simulink model "multirateFilters"  (R2017b)
settings: Solver=FixedStepDiscrete  StartTime=0.0  StopTime=0.02  RelTol=1e-3
undefined symbols (not defined in the file): designMultirateFIR
libraries: dspsrcs4 x4, dsparch4 x2, dspmlti4 x2, dspfdesign x1, dspsigops x1
settings Model: Creator=Lucas  LastModifiedBy=Lucas
settings SolverCC: AutoInsertRateTranBlk=on
settings DataIOCC: LimitDataPoints=on  SaveOutput=off  SignalLogging=off  SaveTime=off
settings OptimizationCC: LifeSpan=inf  SimCompilerOptimization=on
settings DebuggingCC: AlgebraicLoopMsg=error  SingleTaskRateTransMsg=error  AllowSymbolicDim=off  SFUnexpectedBacktrackingDiag=warning  SFNoUnconditionalDefaultTransitionDiag=warning  SFExecutionAtInitializationDiag=none
settings CodeAppCC: StateflowObjectComments=on
settings GRTTargetCC: TargetLangStandard=C89/C90 (ANSI)  GeneratePreprocessorConditionals=Disable all
settings ConfigComp: CovMetricSettings=dw  CovHtmlReporting=on  CovSaveCumulativeToWorkspaceVar=on  CovSaveSingleToWorkspaceVar=on  CovExternalEMLEnable=off  CovSFcnEnable=off

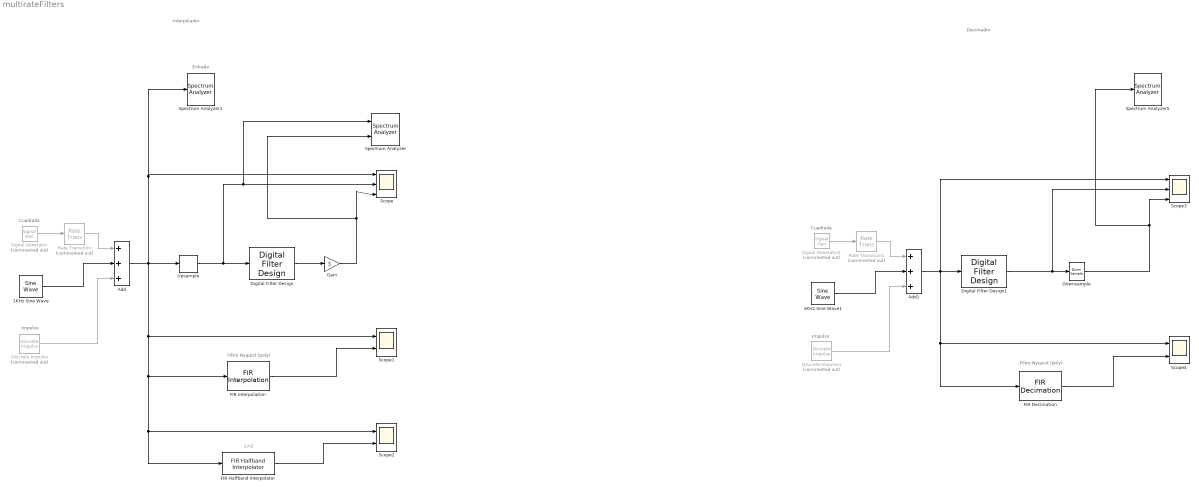
== system multirateFilters ==
  note: Interpolador
  note: Filtro Nyquist (poly)
  note: Entrada
  note: Cuadrada
  note: Filtro Nyquist (poly)
  note: Cuadrada
  note: Decimador
  note: Impulso
  note: Impulso
  note: L=2
  1KHz Sine Wave : dspsrcs4/Sine Wave  Amplitude=1  Frequency=1000  Phase=0  SampleMode=Discrete  OutComplex=Real  CompMethod=Trigonometric fcn  TableSize=Speed  SampleTime=1/10000  SamplesPerFrame=256  ResetState=Restart at time zero  OutputFrames=off  dataType=double  wordLen=16  udDataType=sfix(16)  fracBitsMode=Best precision  numFracBits=15  OutDataTypeStr=double  LastOutDataTypeStr=double
  1KHz Sine Wave1 : dspsrcs4/Sine Wave  Amplitude=1  Frequency=1000  Phase=0  SampleMode=Discrete  OutComplex=Real  CompMethod=Trigonometric fcn  TableSize=Speed  SampleTime=1/10000  SamplesPerFrame=300  ResetState=Restart at time zero  OutputFrames=off  dataType=double  wordLen=16  udDataType=sfix(16)  fracBitsMode=Best precision  numFracBits=15  OutDataTypeStr=double  LastOutDataTypeStr=double
  Add : Sum  Inputs=+++
  Add1 : Sum  Inputs=+++
  Digital Filter Design : dsparch4/Digital Filter Design  mwdsp_browser_bugfix_var=off
  Digital Filter Design1 : dsparch4/Digital Filter Design  mwdsp_browser_bugfix_var=off
  Discrete Impulse : dspsrcs4/Discrete  Impulse  Commented=on  Delay=0  SampleTime=1/10000  FrameSample=256  OutputFrames=off  dataType=double  isSigned=on  wordLen=16  udDataType=sfix(16)  fracBitsMode=Best precision  numFracBits=15  OutDataTypeStr=double  LastOutDataTypeStr=double
  Discrete Impulse1 : dspsrcs4/Discrete  Impulse  Commented=on  Delay=0  SampleTime=1/10000  FrameSample=300  OutputFrames=off  dataType=double  isSigned=on  wordLen=16  udDataType=sfix(16)  fracBitsMode=Best precision  numFracBits=15  OutDataTypeStr=double  LastOutDataTypeStr=double
  Downsample : DownSample  N=3
  FIR Decimation : dspmlti4/FIR Decimation  FilterSource=Auto  h=designMultirateFIR(1,2)  D=3  filtStruct=Direct form  FilterObject=FDECIM  InputProcessing=Columns as channels (frame based)  framing=Enforce single-rate processing  inputOffset=0  outputBufInitCond=0  roundingMode=Floor  overflowMode=off  firstCoeffDataTypeStr=Inherit: Same word length as input  firstCoeffMin=[]  firstCoeffMax=[]  firstCoeffLastDataTypeStr=Inherit: Same word length as input  outputDataTypeStr=Inherit: Same as accumulator  outputMin=[]  outputMax=[]  outputLastDataTypeStr=Inherit: Same as accumulator
  FIR Interpolation : dspmlti4/FIR Interpolation  FilterSource=Auto  h=designMultirateFIR(3,1)  L=3  FilterObject=FINTERP  InputProcessing=Columns as channels (frame based)  framing=Enforce single-rate processing  outputBufInitCond=0  roundingMode=Floor  overflowMode=off  firstCoeffDataTypeStr=Inherit: Same word length as input  firstCoeffMin=[]  firstCoeffMax=[]  firstCoeffLastDataTypeStr=Inherit: Same word length as input  outputDataTypeStr=Inherit: Same as accumulator  outputMin=[]  outputMax=[]  outputLastDataTypeStr=Inherit: Same as accumulator
      settings: SourceProductName=DSP System Toolbox
  FIR Halfband Interpolator : dspfdesign/FIR Halfband Interpolator  Specification=Transition width and stopband attenuation  FilterOrder=52  TransitionWidth=5000  StopbandAttenuation=80  FilterBankInputPort=off  InheritSampleRate=off  SampleRate=10000  SimulateUsing=Code generation  roundingMode=Floor  coeffsDataTypeStr=fixdt(1,16)
      settings: SourceProductName=DSP System Toolbox  SourceProductBaseCode=DS
  Gain : Gain  Gain=3
  Rate Transition : RateTransition  Commented=on
  Rate Transition1 : RateTransition  Commented=on
  Scope : Scope  NumInputPorts=3
  Scope1 : Scope  NumInputPorts=2
  Scope2 : Scope  NumInputPorts=2
  Scope3 : Scope  NumInputPorts=3
  Scope4 : Scope  NumInputPorts=2
  Signal Generator : SignalGenerator  Commented=on  WaveForm=square  Frequency=2000
  Signal Generator1 : SignalGenerator  Commented=on  WaveForm=square  Frequency=2000  Units=rad/sec
  Spectrum Analyzer : SpectrumAnalyzer  NumInputPorts=2
  Spectrum Analyzer1 : SpectrumAnalyzer
  Spectrum Analyzer5 : SpectrumAnalyzer
  Upsample : dspsigops/Upsample  N=3  phase=0  InputProcessing=Columns as channels (frame based)  RateOptions=Enforce single-rate processing  ic=0  mode=Unused parameter value
  wires:
  Add/1 -> Scope1/1, Scope2/1, FIR Halfband Interpolator/1, FIR Interpolation/1, Spectrum Analyzer1/1, Scope/1, Upsample/1
  Upsample/1 -> Spectrum Analyzer/1, Scope/2, Digital Filter Design/1
  FIR Interpolation/1 -> Scope1/2
  Digital Filter Design/1 -> Gain/1
  Gain/1 -> Spectrum Analyzer/2, Scope/3
  1KHz Sine Wave/1 -> Add/2
  Signal Generator/1 -> Rate Transition/1
  Rate Transition/1 -> Add/1
  FIR Halfband Interpolator/1 -> Scope2/2
  Discrete Impulse/1 -> Add/3
  Discrete Impulse1/1 -> Add1/3
  Add1/1 -> Digital Filter Design1/1, Scope4/1, FIR Decimation/1, Scope3/1
  Rate Transition1/1 -> Add1/1
  1KHz Sine Wave1/1 -> Add1/2
  Signal Generator1/1 -> Rate Transition1/1
  FIR Decimation/1 -> Scope4/2
  Downsample/1 -> Spectrum Analyzer5/1, Scope3/3
  Digital Filter Design1/1 -> Scope3/2, Downsample/1
